simulink model "robot_diff_flatness"  (R2013a)
settings: Solver=ode45  StartTime=0.0  StopTime=1000  RelTol=1e-3
InitFcn:
  | param
undefined symbols (not defined in the file or in its folder): ctrl, drawEnvironment, P
settings Model: Creator=beard  LastModifiedBy=beard

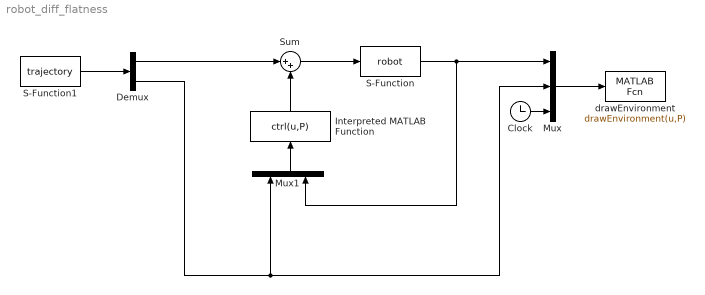
== system robot_diff_flatness ==
  Clock : Clock
  Demux : Demux  Outputs=[2;4]
  Interpreted MATLAB Function : MATLABFcn  MATLABFcn=ctrl(u,P)  OutputDimensions=2  SampleTime=.01
  Mux : Mux  Inputs=3
  Mux1 : Mux  Inputs=2
  S-Function : S-Function  FunctionName=robot  Parameters=P  EnableBusSupport=off
  S-Function1 : S-Function  FunctionName=trajectory  Parameters=P  EnableBusSupport=off
  Sum : Sum  Inputs=|++
  drawEnvironment : MATLABFcn  MATLABFcn=drawEnvironment(u,P)  OutputDimensions=0  SampleTime=.1
  wires:
  S-Function1/1 -> Demux/1
  Clock/1 -> Mux/3
  S-Function/1 -> Mux1/2, Mux/1
  Mux/1 -> drawEnvironment/1
  Demux/2 -> Mux/2, Mux1/1
  Sum/1 -> S-Function/1
  Demux/1 -> Sum/1
  Interpreted MATLAB Function/1 -> Sum/2
  Mux1/1 -> Interpreted MATLAB Function/1
